simulink model "figure_1_5"  (R2026a)
settings: Solver=ode5  FixedStep=1e-4
settings Model: Creator=yagmu  LastModifiedBy=yagmu

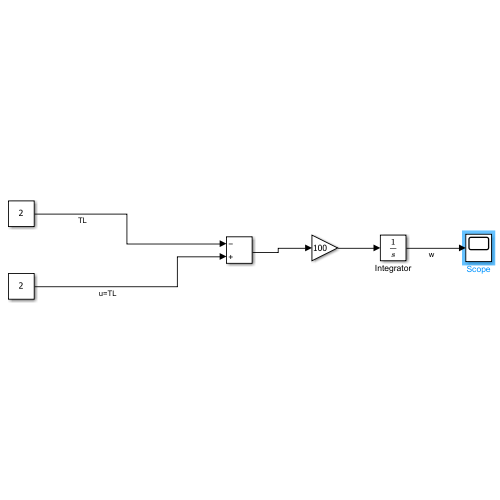
[thumbnail: Simulink's stored preview of the top-level diagram]
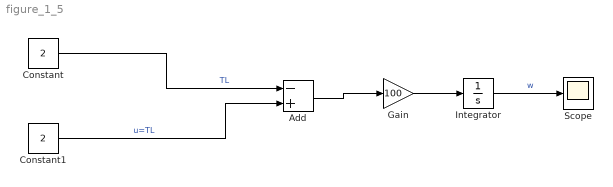
== system figure_1_5 ==
  Add : Sum  Inputs=-+
  Constant : Constant  Value=2
  Constant1 : Constant  Value=2
  Gain : Gain  Gain=100
  Integrator : Integrator
  Scope : Scope
      settings: ActiveDisplayYMinimum=-1  ActiveDisplayYMaximum=1
  wires:
  Constant/1 -> Add/1  "TL"
  Constant1/1 -> Add/2  "u=TL"
  Add/1 -> Gain/1
  Gain/1 -> Integrator/1
  Integrator/1 -> Scope/1  "w"
